simulink model "acc_sim"  (R2024a)
settings: Solver=ode4  StartTime=0.0  StopTime=inf  RelTol=1e-3
undefined symbols (not defined in the file or in its folder): K_d, K_i, K_p
libraries: canoelib x9, simulink x4
settings Model: Creator=Administrator  LastModifiedBy=user
settings DebuggingCC: UnconnectedInputMsg=warning  UnconnectedOutputMsg=warning  UnconnectedLineMsg=warning
settings ModelReferenceCC: EnableRefExpFcnMdlSchedulingChecks=on
settings RTWCC: GPUComputeCapability=3.5  DLArmComputeVersion=19.05

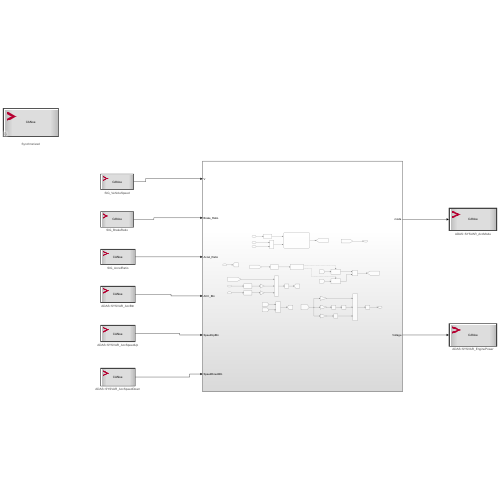
[thumbnail: Simulink's stored preview of the top-level diagram]
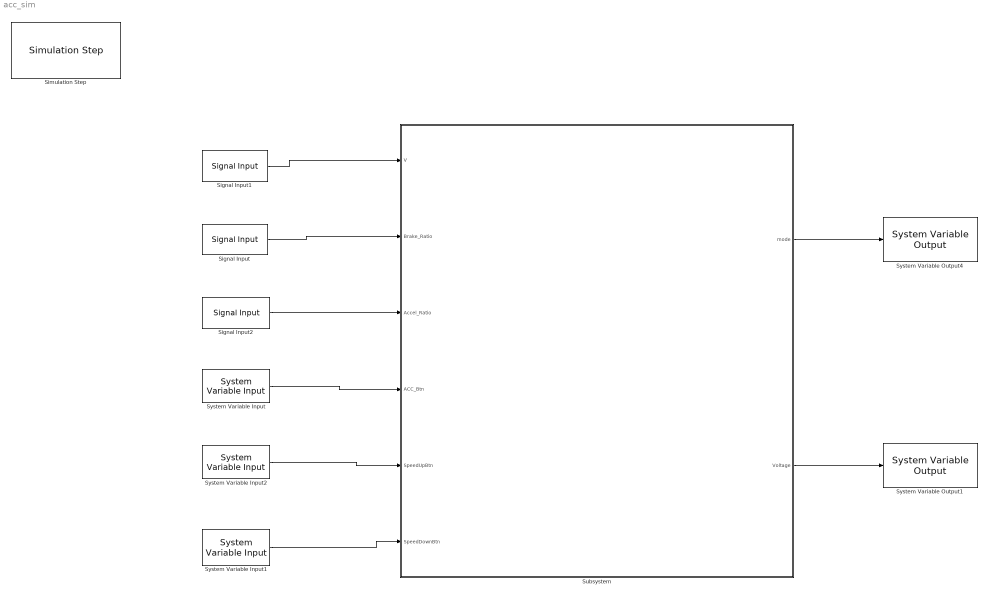
== system acc_sim ==
  Signal Input : canoelib/CANoe I//O/Signal Input  dbName=ACC_DB  nodeName=GatewayA  msgName=MSG_BreakPadel  sigName=SIG_BrakeRatio  editSampleTime=0  rawValue=Default  dataType=uint8  dataTypeDB=uint8  hasEncoding=off
      settings: AttributesFormatString=%<sigName>  SourceProductName=Vector CANoe
  Signal Input1 : canoelib/CANoe I//O/Signal Input  dbName=ACC_DB  nodeName=GatewayA  msgName=MSG_ReadlSpeed  sigName=SIG_VehicleSpeed  editSampleTime=0  rawValue=Default  dataType=int16  dataTypeDB=uint8  hasEncoding=off
      settings: AttributesFormatString=%<sigName>  SourceProductName=Vector CANoe
  Signal Input2 : canoelib/CANoe I//O/Signal Input  dbName=ACC_DB  nodeName=GatewayA  msgName=MSG_AccelPadel  sigName=SIG_AccelRatio  editSampleTime=0  rawValue=Default  dataType=uint8  dataTypeDB=uint8  hasEncoding=off
      settings: AttributesFormatString=%<sigName>  SourceProductName=Vector CANoe
  Simulation Step : canoelib/CANoe I//O/Simulation Step  mode=Synchronized
      settings: AttributesFormatString=%<mode>  SourceProductName=Vector CANoe
  Subsystem : Subsystem
  System Variable Input : canoelib/CANoe I//O/System Variable Input  nsName=ADAS  sysVarName=SYSVAR_AccBtn  arrayIndex=-1  editSampleTime=0  rawValue=Default  dataType=Default  dataTypeDB=uint32  hasEncoding=off  dataTypeCANoe=Get from CANoe
      settings: AttributesFormatString=%<nsName>::%<sysVarName>  SourceProductName=Vector CANoe
  System Variable Input1 : canoelib/CANoe I//O/System Variable Input  nsName=ADAS  sysVarName=SYSVAR_AccSpeedDown  arrayIndex=-1  editSampleTime=0  rawValue=Default  dataType=Default  dataTypeDB=uint32  hasEncoding=off  dataTypeCANoe=Get from CANoe
      settings: AttributesFormatString=%<nsName>::%<sysVarName>  SourceProductName=Vector CANoe
  System Variable Input2 : canoelib/CANoe I//O/System Variable Input  nsName=ADAS  sysVarName=SYSVAR_AccSpeedUp  arrayIndex=-1  editSampleTime=0  rawValue=Default  dataType=Default  dataTypeDB=uint32  hasEncoding=off  dataTypeCANoe=Get from CANoe
      settings: AttributesFormatString=%<nsName>::%<sysVarName>  SourceProductName=Vector CANoe
  System Variable Output1 : canoelib/CANoe I//O/System Variable Output  nsName=ADAS  sysVarName=SYSVAR_EnginePower  arrayIndex=-1  rawValue=Default  dataType=double  dataTypeDB=double  hasEncoding=off  dataTypeCANoe=Get from CANoe
      settings: AttributesFormatString=%<nsName>::%<sysVarName>  SourceProductName=Vector CANoe
  System Variable Output4 : canoelib/CANoe I//O/System Variable Output  nsName=ADAS  sysVarName=SYSVAR_AccMode  arrayIndex=-1  rawValue=Default  dataType=uint32  dataTypeDB=uint32  hasEncoding=off  dataTypeCANoe=Get from CANoe
      settings: AttributesFormatString=%<nsName>::%<sysVarName>  SourceProductName=Vector CANoe
  wires:
  Subsystem/1(mode) -> System Variable Output4/1
  Signal Input/1 -> Subsystem/2(Brake_Ratio)
  Signal Input2/1 -> Subsystem/3(Accel_Ratio)
  Signal Input1/1 -> Subsystem/1(V)
  System Variable Input/1 -> Subsystem/4(ACC_Btn)
  System Variable Input1/1 -> Subsystem/6(SpeedDownBtn)
  System Variable Input2/1 -> Subsystem/5(SpeedUpBtn)
  Subsystem/2(Voltage) -> System Variable Output1/1

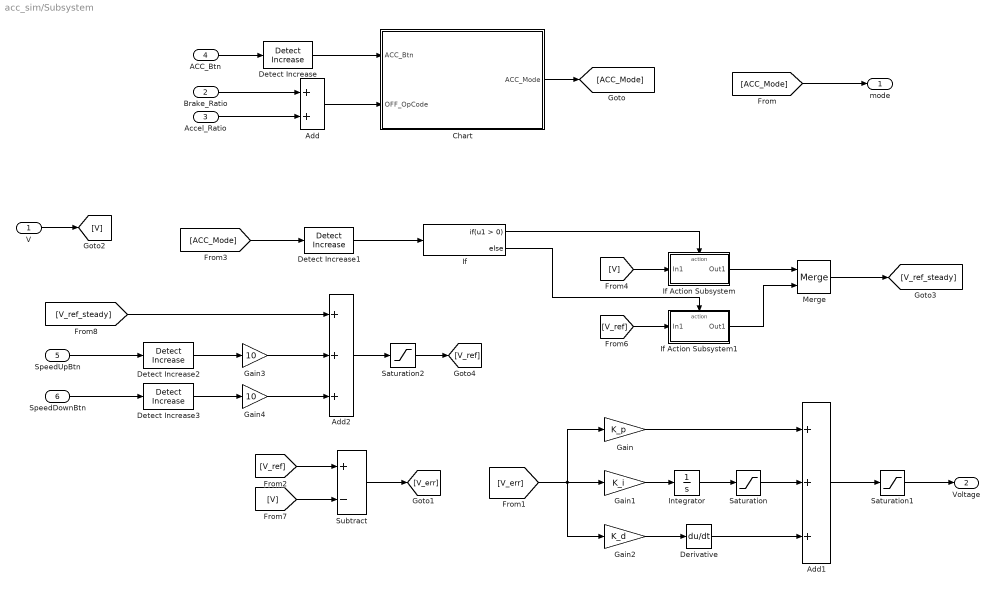
== system acc_sim/Subsystem ==
  V : Inport
  Brake_Ratio : Inport  Port=2
  Accel_Ratio : Inport  Port=3
  ACC_Btn : Inport  Port=4
  SpeedUpBtn : Inport  Port=5
  SpeedDownBtn : Inport  Port=6
  Add : Sum
  Add1 : Sum  Inputs=+++
  Add2 : Sum  Inputs=+++
  Chart : Stateflow chart  TreatAsAtomicUnit=on
  Derivative : Derivative
  Detect Increase{,1..3} (4 alike) : simulink/Logic and Bit Operations/Detect Increase  vinit=0.0  OutDataTypeStr=boolean
  Gain : Gain  Gain=K_p
  Gain1 : Gain  Gain=K_i
  Gain2 : Gain  Gain=K_d
  Gain3 : Gain  Gain=10
  Gain4 : Gain  Gain=10
  If : If
  If Action Subsystem : Subsystem  TreatAsAtomicUnit=on
  If Action Subsystem1 : Subsystem  TreatAsAtomicUnit=on
  Integrator : Integrator
  Merge : Merge
  Saturation : Saturate  UpperLimit=78  LowerLimit=0
  Saturation1 : Saturate  UpperLimit=78  LowerLimit=0
  Saturation2 : Saturate  UpperLimit=250  LowerLimit=0
  Subtract : Sum  Inputs=+-
  mode : Outport
  Voltage : Outport  Port=2
  wires:
  ACC_Btn/1 -> Detect Increase/1
  Brake_Ratio/1 -> Add/1
  Accel_Ratio/1 -> Add/2
  Add/1 -> Chart/2(OFF_OpCode)
  Subtract/1 -> [V_err]
  [V_err] -> Gain/1, Gain1/1, Gain2/1
  Gain1/1 -> Integrator/1
  Gain/1 -> Add1/1
  Gain2/1 -> Derivative/1
  Integrator/1 -> Saturation/1
  Derivative/1 -> Add1/3
  Saturation/1 -> Add1/2
  Add1/1 -> Saturation1/1
  Saturation1/1 -> Voltage/1
  Detect Increase/1 -> Chart/1(ACC_Btn)
  Chart/1(ACC_Mode) -> [ACC_Mode]
  [ACC_Mode] -> mode/1
  [ACC_Mode] -> Detect Increase1/1
  Detect Increase1/1 -> If/1
  V/1 -> [V]
  [V] -> If Action Subsystem/1(In1)
  If/1 -> If Action Subsystem/Action
  If/2 -> If Action Subsystem1/Action
  [V_ref] -> If Action Subsystem1/1(In1)
  If Action Subsystem/1(Out1) -> Merge/1
  If Action Subsystem1/1(Out1) -> Merge/2
  Merge/1 -> [V_ref_steady]
  SpeedDownBtn/1 -> Detect Increase3/1
  SpeedUpBtn/1 -> Detect Increase2/1
  [V_ref] -> Subtract/1
  [V] -> Subtract/2
  Detect Increase2/1 -> Gain3/1
  Detect Increase3/1 -> Gain4/1
  [V_ref_steady] -> Add2/1
  Gain3/1 -> Add2/2
  Gain4/1 -> Add2/3
  Add2/1 -> Saturation2/1
  Saturation2/1 -> [V_ref]

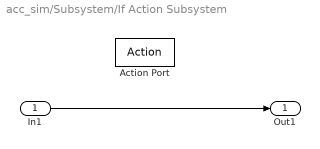
== system acc_sim/Subsystem/If Action Subsystem ==
  In1 : Inport
  Action Port : ActionPort  ActionPortLabel=if(u1 > 0)
  Out1 : Outport
  wires:
  In1/1 -> Out1/1

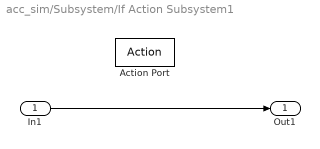
== system acc_sim/Subsystem/If Action Subsystem1 ==
  In1 : Inport
  Action Port : ActionPort  ActionPortLabel=else
  Out1 : Outport
  wires:
  In1/1 -> Out1/1

== stateflow chart acc_sim/Subsystem/Chart ==
  state ACC_On
    ACC_Mode = 1;
  state ACC_Off
    ACC_Mode = 0;
  ACC_Off -> ACC_On : [ACC_Btn == 1]
  (default) -> ACC_Off
  ACC_On -> ACC_Off : [ACC_Btn == 1 || OFF_OpCode > 0]
  data: ACC_Btn input; ACC_Mode output; OFF_OpCode input
